simulink model "series_RC"  (R2019a)
settings: Solver=VariableStepAuto  StartTime=0.0  StopTime=0.05  RelTol=1e-3
settings Model: Creator=anubh  LastModifiedBy=anubh

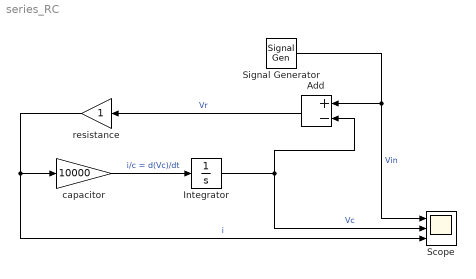
== system series_RC ==
  Add : Sum  Inputs=+-
  Integrator : Integrator
  Scope : Scope  NumInputPorts=3
  Signal Generator : SignalGenerator  WaveForm=square  Amplitude=5  Frequency=1000
  capacitor : Gain  Gain=10000
  resistance : Gain
  wires:
  Integrator/1 -> Scope/2, Add/2  "Vc"
  capacitor/1 -> Integrator/1  "i/c = d(Vc)/dt"
  resistance/1 -> capacitor/1, Scope/3  "i"
  Add/1 -> resistance/1  "Vr"
  Signal Generator/1 -> Add/1, Scope/1  "Vin"
